simulink model "convex_combi_receiver"  (R2023b)
settings: Solver=FixedStepAuto  StartTime=0.0  StopTime=10.0  RelTol=1e-3
undefined symbols (not defined in the file): DiscIntNeverNeededParam
libraries: dspstat3 x8, dspadpt3 x4, androidaudiovideolib x1, fuzblock x1, androidcommunicationlib x1
settings Model: Creator=Asus  LastModifiedBy=Asus
settings OptimizationCC: EnhancedBackFolding=on  PassReuseOutputArgsAs=Individual arguments  ZeroExternalMemoryAtStartup=off  ZeroInternalMemoryAtStartup=off  MaxStackSize=64  OptimizeBlockOrder=speed  DifferentSizesBufferReuse=on  OptimizationCustomize=off  EfficientTunableParamExpr=on
settings DebuggingCC: ParameterTunabilityLossMsg=error
settings HardwareCC: ProdBitPerLong=64  ProdLargestAtomicInteger=LongLong  ProdLargestAtomicFloat=Double  ProdLongLongMode=on  ProdHWDeviceType=ARM Compatible->ARM 64-bit (LP64)
settings SFSimCC: MATLABDynamicMemAlloc=off
settings RTWCC: Description=Embedded Coder  SystemTargetFile=ert.tlc  HardwareBoard=Android Device (64bit)  TLCOptions="-aInlineSetEventsForThisBaseRateFcn=TLC_FALSE -aSuppressMultiTaskScheduler=TLC_FALSE  -aRateBasedStepFcn=0"  TemplateMakefile=ert_default_tmf  RTWVerbose=off  Toolchain=Android SDK/NDK Tools
settings CodeAppCC: ForceParamTrailComments=on  IgnoreCustomStorageClasses=off  OperatorAnnotations=on  SimulinkDataObjDesc=on  SFDataObjDesc=on  InsertBlockDesc=on

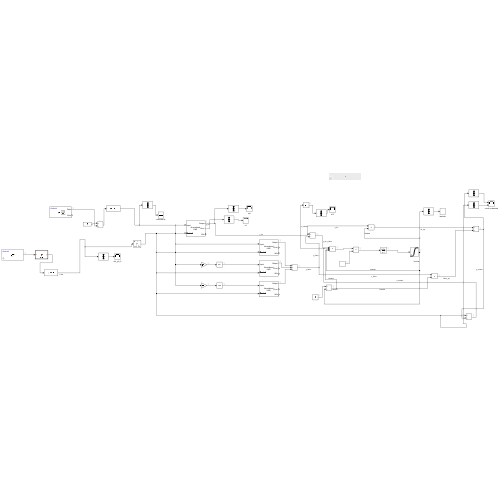
[thumbnail: Simulink's stored preview of the top-level diagram]
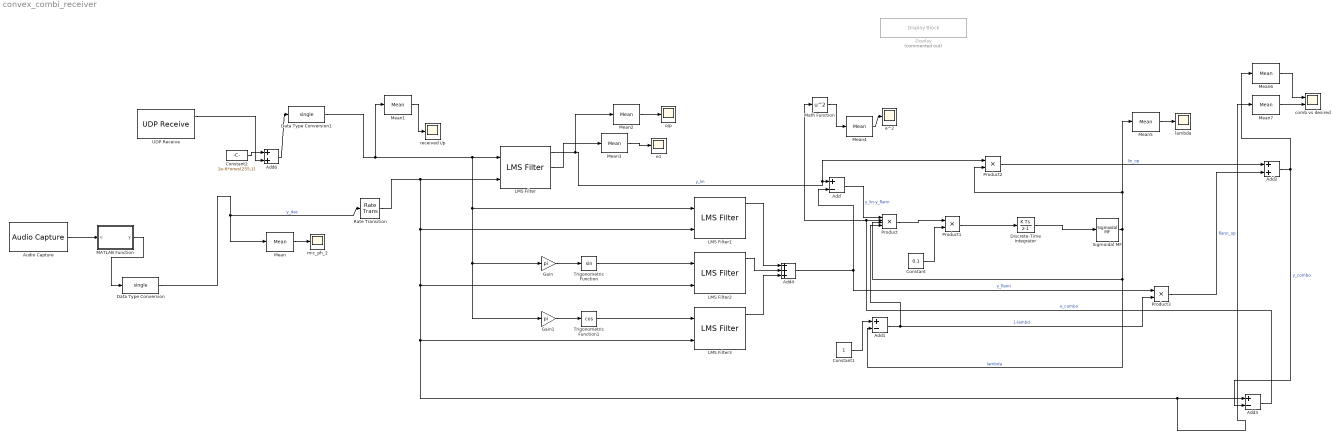
== system convex_combi_receiver ==
  Add : Sum  Inputs=+-
  Add1 : Sum  Inputs=+-
  Add2 : Sum
  Add3 : Sum  Inputs=+-
  Add4 : Sum  Inputs=+++
  Add6 : Sum
  Audio Capture : androidaudiovideolib/Audio Capture  SampleFreq=16000  FrameSize=255  SampleTime=0.015938  SimulateUsing=Code generation  DeviceStr=0  QueueDuration=0  BlockPlatform=Android  AudioSamplingFreq=44100
  Constant : Constant  Value=0.1
  Constant1 : Constant
  Constant2 : Constant  Value=1e-6*ones(255,1)  OutDataTypeStr=single
  Data Type Conversion : DataTypeConversion  OutDataTypeStr=single  SaturateOnIntegerOverflow=off  RndMeth=Floor
  Data Type Conversion1 : DataTypeConversion  OutDataTypeStr=single  SaturateOnIntegerOverflow=off  RndMeth=Floor
  Discrete-Time Integrator : DiscreteIntegrator  SampleTime=-1  ICPrevOutput=DiscIntNeverNeededParam  ICPrevScaledInput=DiscIntNeverNeededParam
  Display : DisplayBlock  Commented=on  LabelPosition=Hide  Transparency=1
  Gain : Gain  Gain=pi
  Gain1 : Gain  Gain=pi
  LMS Filter : dspadpt3/LMS Filter  Algo=Normalized LMS  L=4  stepflag=Dialog  mu=0.1  leakage=1.0  ic=0  Adapt=off  resetflag=None  weights=on  addnparflag=off  roundingMode=Floor  overflowMode=on  firstCoeffMode=Specify word length  firstCoeffWordLength=16  firstCoeffFracLength=15
  LMS Filter1 : dspadpt3/LMS Filter  Algo=Normalized LMS  L=96  stepflag=Dialog  mu=0.001  leakage=1.0  ic=0  Adapt=off  resetflag=None  weights=on  addnparflag=off  roundingMode=Floor  overflowMode=off
  LMS Filter2 : dspadpt3/LMS Filter  Algo=Normalized LMS  L=96  stepflag=Dialog  mu=0.001  leakage=1.0  ic=0  Adapt=off  resetflag=None  weights=on  addnparflag=off  roundingMode=Floor  overflowMode=off
  LMS Filter3 : dspadpt3/LMS Filter  Algo=Normalized LMS  L=96  stepflag=Dialog  mu=0.001  leakage=1.0  ic=0  Adapt=off  resetflag=None  weights=on  addnparflag=off  roundingMode=Floor  overflowMode=off
  MATLAB Function : MATLAB Function  TreatAsAtomicUnit=on
  Math Function : Math  Operator=square
  Mean{,1..7} (8 alike) : dspstat3/Mean  run=off  InputProcessing=Columns as channels (frame based)  reset_popup=None  directionMode=Entire input  dimension=1  roiEnable=off  roiType=Rectangles  roiPortion=Entire ROI  roiOutput=Individual statistics for each ROI  roiFlag=off  roundingMode=Floor  overflowMode=off  outputDataTypeStr=Inherit: Same as accumulator  outputMin=[]  outputMax=[]  outputLastDataTypeStr=Inherit: Same as accumulator
  Product : Product  Inputs=4
  Product1 : Product
  Product2 : Product
  Product3 : Product
  Rate Transition : RateTransition  Integrity=off  OutPortSampleTimeOpt=Inherit
  Sigmoidal MF : fuzblock/Membership  Functions/Sigmoidal MF  a=1  c=0
  Trigonometric Function : Trigonometry
  Trigonometric Function1 : Trigonometry  Operator=cos
  UDP Receive : androidcommunicationlib/UDP Receive  localURL='0.0.0.0'  localPort=25000  remoteURL='0.0.0.0'  remotePort=-1  recvBufferSize=8192  signalDatatype=single  dims=255  isVarSize=off  showBlockingTime=off  blockingTime=0  sampletime=255/16000  blockPlatform=Android
  comb vs desired : Scope  NumInputPorts=2
  e1 : Scope
  e^2 : Scope
  lambda : Scope
  mic_ph_2 : Scope
  o/p : Scope
  received i/p : Scope
  wires:
  LMS Filter/1 -> Mean2/1, Product2/1, Add/1  "y_lin"
  Rate Transition/1 -> LMS Filter/2, Mean7/1, Add3/1, LMS Filter3/2, LMS Filter2/2, LMS Filter1/2
  LMS Filter/2 -> Mean3/1
  Product2/1 -> Add2/1  "lin_op"
  Add4/1 -> Add/2, Product3/1  "y_flann"
  Audio Capture/1 -> MATLAB Function/1(u)
  UDP Receive/1 -> Add6/2
  LMS Filter3/1 -> Add4/3
  Data Type Conversion/1 -> Mean/1, Rate Transition/1  "y_des"
  Sigmoidal MF/1 -> Mean5/1, Product2/2, Add1/2, Product/3  "lambda"
  Add1/1 -> Product/4, Product3/2  "1-lambd"
  Discrete-Time Integrator/1 -> Sigmoidal MF/1
  Add/1 -> Product/1  "y_lin-y_flann"
  Trigonometric Function1/1 -> LMS Filter3/1
  Gain/1 -> Trigonometric Function/1
  Add6/1 -> Data Type Conversion1/1
  Trigonometric Function/1 -> LMS Filter2/1
  Constant1/1 -> Add1/1
  Gain1/1 -> Trigonometric Function1/1
  Product3/1 -> Add2/2  "flann_op"
  Data Type Conversion1/1 -> Mean1/1, LMS Filter/1, LMS Filter1/1, Gain1/1, Gain/1
  Add3/1 -> Math Function/1, Product/2  "e_combo"
  Add2/1 -> Mean6/1, Add3/2  "y_combo"
  LMS Filter1/1 -> Add4/1
  Math Function/1 -> Mean4/1
  Product/1 -> Product1/1
  LMS Filter2/1 -> Add4/2
  Product1/1 -> Discrete-Time Integrator/1
  MATLAB Function/1(y) -> Data Type Conversion/1
  Constant/1 -> Product1/2
  Constant2/1 -> Add6/1
  Mean/1 -> mic_ph_2/1
  Mean1/1 -> received i/p/1
  Mean2/1 -> o/p/1
  Mean3/1 -> e1/1
  Mean4/1 -> e^2/1
  Mean5/1 -> lambda/1
  Mean7/1 -> comb vs desired/2
  Mean6/1 -> comb vs desired/1

== matlab function convex_combi_receiver/MATLAB Function ==
  data: u input; y output
function y = fcn(u)
    % u is [64x2] (Left and Right channels)
    % y is [64x1] (Mono output - Left channel)
    
    y = u(:, 1); % Extract only the first column
end
